simulink model "ThdRwLtStCshnFldIsPosChk1"  (R2024b)
settings: Solver=FixedStepDiscrete  StartTime=0.0  StopTime=10.0  FixedStep=0.01  RelTol=1e-3
undefined symbols (not defined in the file or in its folder): KeSMSuThrdRwCushFoldPosDelta_Val, KeSMSuThrdRwCushFoldPosTolr_Val
libraries: StIsPosChkLib x8, simulink x5
settings Model: Creator=sn2xws  LastModifiedBy=sn55gm
settings Model: ModifiedHistory=|
  | 2024.3.14
  | V2.3.0
  | Bug 813950 童锁Lock，Mode1_Easy Entry Mode 不应调用失败
  | 2024.6.25
  | V3.0.0 557模式流程V1.6
  | 2024.9.6 V3.0.1 新增Md56
  | 2024.10.14 V3.0.2 Md56使用的标定值修正
  | 2025.12.19 V3.8.0 Bug 991386 Md1 三排占座时未移动且报了成功
  | 2025.7.1 V3.13.0 新增MD61 MD62
settings SolverCC: AlgebraicLoopSolver=TrustRegion
settings DataIOCC: SaveFormat=StructureWithTime  ReturnWorkspaceOutputs=off
settings OptimizationCC: DefaultParameterBehavior=Inlined  EnhancedBackFolding=on  PassReuseOutputArgsAs=Individual arguments  ZeroExternalMemoryAtStartup=off  ZeroInternalMemoryAtStartup=off  OptimizeBlockOrder=speed  DifferentSizesBufferReuse=on  OptimizationCustomize=off  EfficientTunableParamExpr=on
settings DebuggingCC: ParameterTunabilityLossMsg=error  UnconnectedInputMsg=warning  UnconnectedOutputMsg=warning  UnconnectedLineMsg=warning  ArithmeticOperatorsInVariantConditions=warning
settings ModelReferenceCC: EnableRefExpFcnMdlSchedulingChecks=on  ModelReferenceNumInstancesAllowed=Single
settings SFSimCC: MATLABDynamicMemAlloc=off  CustomCodeUndefinedFunction=UseInterfaceOnly
settings RTWCC: Description=AUTOSAR  SystemTargetFile=autosar.tlc  GenCodeOnly=on  TemplateMakefile=ert_default_tmf  GenerateReport=on  IncludeHyperlinkInReport=on  LaunchReport=on  DataTypeReplacement=CDataTypesFixedWidth  GenerateTraceInfo=on  GenerateTraceReport=on  GenerateTraceReportSl=on  GenerateTraceReportSf=on  GenerateTraceReportEml=on  GPUComputeCapability=3.5
settings CodeAppCC: ForceParamTrailComments=on  IgnoreCustomStorageClasses=off  OperatorAnnotations=on  SimulinkDataObjDesc=on  SFDataObjDesc=on  InsertBlockDesc=on
settings STFCustomTargetCC: TargetLangStandard=C99 (ISO)  MultiwordLength=256  ParMdlRefBuildCompliant=on  CompOptLevelCompliant=on  IncludeMdlTerminateFcn=off  CombineOutputUpdateFcns=on  SuppressErrorStatus=on  ERTCustomFileBanners=on  SupportNonFinite=off  SupportComplex=off  SupportContinuousTime=off  SupportNonInlinedSFcns=off  RemoveResetFunc=on  MATLABClassNameForMDSCustomization=Simulink.SoftwareTarget.ERTCustomization  AutosarCompliant=on  UseToolchainInfoCompliant=on  LookupTableObjectStructAxisOrder=2,1,3,4,...  LUTObjectStructOrderEvenSpacing=Size,Table,Breakpoints  SystemTargetFile=autosar.tlc
settings ERTTargetCC: TargetLangStandard=C99 (ISO)  ConcurrentExecutionCompliant=off  IncludeMdlTerminateFcn=off  SuppressErrorStatus=on  SupportNonFinite=off  SupportComplex=off  ModelStepFunctionPrototypeControlCompliant=off  CPPClassGenCompliant=off  AutosarCompliant=on  LookupTableObjectStructAxisOrder=2,1,3,4,...  LUTObjectStructOrderEvenSpacing=Size,Table,Breakpoints  ERTCustomFileTemplate=example_file_process.tlc  ERTFilePackagingFormat=Compact  BooleanTrueId=TRUE  BooleanFalseId=FALSE  DynamicArrayContainerType=coder::array

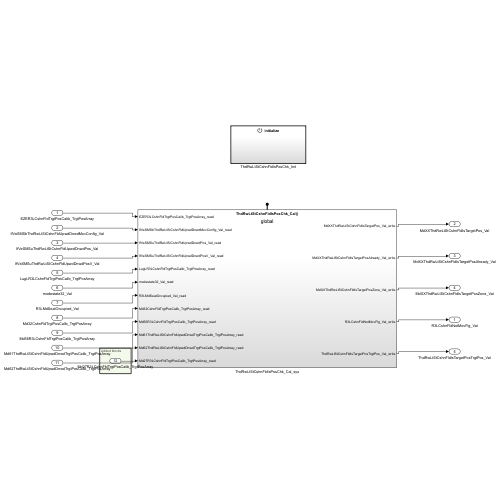
[thumbnail: Simulink's stored preview of the top-level diagram]
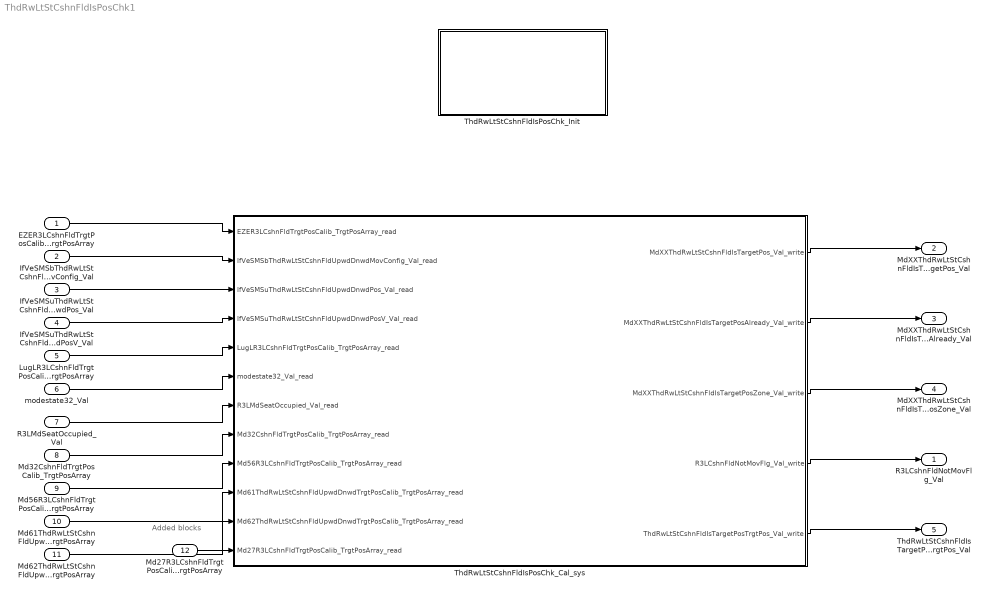
== system ThdRwLtStCshnFldIsPosChk1 ==
  note: Added blocks
  EZER3LCshnFldTrgtPosCalib_TrgtPosArray : Inport  Description=|  OutDataTypeStr=uint16  PortDimensions=3
      | 0:Pos
      | 1:Max
      | 2:Min
  IfVeSMSbThdRwLtStCshnFldUpwdDnwdMovConfig_Val : Inport  Port=2  OutDataTypeStr=boolean  PortDimensions=1
  IfVeSMSuThdRwLtStCshnFldUpwdDnwdPos_Val : Inport  Port=3  OutDataTypeStr=uint16  PortDimensions=1
  IfVeSMSuThdRwLtStCshnFldUpwdDnwdPosV_Val : Inport  Port=4  OutDataTypeStr=boolean  PortDimensions=1
  LugLR3LCshnFldTrgtPosCalib_TrgtPosArray : Inport  Description=|  Port=5  OutDataTypeStr=uint16  PortDimensions=3
      | 0:Pos
      | 1:Max
      | 2:Min
  modestate32_Val : Inport  Port=6  OutDataTypeStr=uint32  PortDimensions=1
  R3LMdSeatOccupied_Val : Inport  Port=7  OutDataTypeStr=boolean  PortDimensions=1
  Md32CshnFldTrgtPosCalib_TrgtPosArray : Inport  Description=|  Port=8  OutDataTypeStr=uint16  PortDimensions=3
      | 0:Pos
      | 1:Max
      | 2:Min
  Md56R3LCshnFldTrgtPosCalib_TrgtPosArray : Inport  Description=|  Port=9  OutDataTypeStr=uint16  PortDimensions=3
      | 0:Pos
      | 1:Max
      | 2:Min
  Md61ThdRwLtStCshnFldUpwdDnwdTrgtPosCalib_TrgtPosArray : Inport  Description=|  Port=10  OutDataTypeStr=uint16  PortDimensions=3
      | 0:Pos
      | 1:Max
      | 2:Min
  Md62ThdRwLtStCshnFldUpwdDnwdTrgtPosCalib_TrgtPosArray : Inport  Description=|  Port=11  OutDataTypeStr=uint16  PortDimensions=3
      | 0:Pos
      | 1:Max
      | 2:Min
  Md27R3LCshnFldTrgtPosCalib_TrgtPosArray : Inport  Description=|  Port=12  OutDataTypeStr=uint16  PortDimensions=3
      | 0:Pos
      | 1:Max
      | 2:Min
  ThdRwLtStCshnFldIsPosChk_Cal_sys : Subsystem
  ThdRwLtStCshnFldIsPosChk_Init : Subsystem
  R3LCshnFldNotMovFlg_Val : Outport  OutDataTypeStr=boolean  PortDimensions=1  VectorParamsAs1DForOutWhenUnconnected=off
  MdXXThdRwLtStCshnFldIsTargetPos_Val : Outport  Port=2  OutDataTypeStr=uint32  PortDimensions=1  VectorParamsAs1DForOutWhenUnconnected=off
  MdXXThdRwLtStCshnFldIsTargetPosAlready_Val : Outport  Port=3  OutDataTypeStr=uint32  PortDimensions=1  VectorParamsAs1DForOutWhenUnconnected=off
  MdXXThdRwLtStCshnFldIsTargetPosZone_Val : Outport  Port=4  OutDataTypeStr=uint32  PortDimensions=1  VectorParamsAs1DForOutWhenUnconnected=off
  ThdRwLtStCshnFldIsTargetPosTrgtPos_Val : Outport  Port=5  OutDataTypeStr=uint16  PortDimensions=1  VectorParamsAs1DForOutWhenUnconnected=off
  wires:
  EZER3LCshnFldTrgtPosCalib_TrgtPosArray/1 -> ThdRwLtStCshnFldIsPosChk_Cal_sys/1(EZER3LCshnFldTrgtPosCalib_TrgtPosArray_read)
  IfVeSMSbThdRwLtStCshnFldUpwdDnwdMovConfig_Val/1 -> ThdRwLtStCshnFldIsPosChk_Cal_sys/2(IfVeSMSbThdRwLtStCshnFldUpwdDnwdMovConfig_Val_read)
  IfVeSMSuThdRwLtStCshnFldUpwdDnwdPos_Val/1 -> ThdRwLtStCshnFldIsPosChk_Cal_sys/3(IfVeSMSuThdRwLtStCshnFldUpwdDnwdPos_Val_read)
  IfVeSMSuThdRwLtStCshnFldUpwdDnwdPosV_Val/1 -> ThdRwLtStCshnFldIsPosChk_Cal_sys/4(IfVeSMSuThdRwLtStCshnFldUpwdDnwdPosV_Val_read)
  LugLR3LCshnFldTrgtPosCalib_TrgtPosArray/1 -> ThdRwLtStCshnFldIsPosChk_Cal_sys/5(LugLR3LCshnFldTrgtPosCalib_TrgtPosArray_read)
  modestate32_Val/1 -> ThdRwLtStCshnFldIsPosChk_Cal_sys/6(modestate32_Val_read)
  ThdRwLtStCshnFldIsPosChk_Cal_sys/1(MdXXThdRwLtStCshnFldIsTargetPos_Val_write) -> MdXXThdRwLtStCshnFldIsTargetPos_Val/1
  ThdRwLtStCshnFldIsPosChk_Cal_sys/2(MdXXThdRwLtStCshnFldIsTargetPosAlready_Val_write) -> MdXXThdRwLtStCshnFldIsTargetPosAlready_Val/1
  ThdRwLtStCshnFldIsPosChk_Cal_sys/3(MdXXThdRwLtStCshnFldIsTargetPosZone_Val_write) -> MdXXThdRwLtStCshnFldIsTargetPosZone_Val/1
  ThdRwLtStCshnFldIsPosChk_Cal_sys/4(R3LCshnFldNotMovFlg_Val_write) -> R3LCshnFldNotMovFlg_Val/1
  ThdRwLtStCshnFldIsPosChk_Cal_sys/5(ThdRwLtStCshnFldIsTargetPosTrgtPos_Val_write) -> ThdRwLtStCshnFldIsTargetPosTrgtPos_Val/1
  R3LMdSeatOccupied_Val/1 -> ThdRwLtStCshnFldIsPosChk_Cal_sys/7(R3LMdSeatOccupied_Val_read)
  Md32CshnFldTrgtPosCalib_TrgtPosArray/1 -> ThdRwLtStCshnFldIsPosChk_Cal_sys/8(Md32CshnFldTrgtPosCalib_TrgtPosArray_read)
  Md56R3LCshnFldTrgtPosCalib_TrgtPosArray/1 -> ThdRwLtStCshnFldIsPosChk_Cal_sys/9(Md56R3LCshnFldTrgtPosCalib_TrgtPosArray_read)
  Md61ThdRwLtStCshnFldUpwdDnwdTrgtPosCalib_TrgtPosArray/1 -> ThdRwLtStCshnFldIsPosChk_Cal_sys/10(Md61ThdRwLtStCshnFldUpwdDnwdTrgtPosCalib_TrgtPosArray_read)
  Md62ThdRwLtStCshnFldUpwdDnwdTrgtPosCalib_TrgtPosArray/1 -> ThdRwLtStCshnFldIsPosChk_Cal_sys/11(Md62ThdRwLtStCshnFldUpwdDnwdTrgtPosCalib_TrgtPosArray_read)
  Md27R3LCshnFldTrgtPosCalib_TrgtPosArray/1 -> ThdRwLtStCshnFldIsPosChk_Cal_sys/12(Md27R3LCshnFldTrgtPosCalib_TrgtPosArray_read)

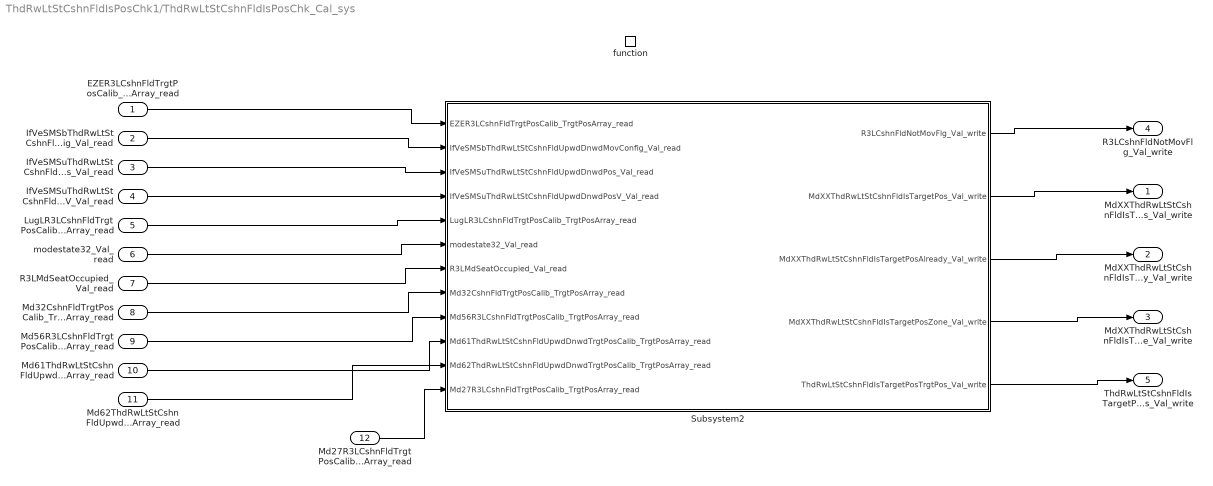
== system ThdRwLtStCshnFldIsPosChk1/ThdRwLtStCshnFldIsPosChk_Cal_sys ==
  EZER3LCshnFldTrgtPosCalib_TrgtPosArray_read : Inport
  IfVeSMSbThdRwLtStCshnFldUpwdDnwdMovConfig_Val_read : Inport  Port=2
  IfVeSMSuThdRwLtStCshnFldUpwdDnwdPos_Val_read : Inport  Port=3
  IfVeSMSuThdRwLtStCshnFldUpwdDnwdPosV_Val_read : Inport  Port=4
  LugLR3LCshnFldTrgtPosCalib_TrgtPosArray_read : Inport  Port=5
  modestate32_Val_read : Inport  Port=6
  R3LMdSeatOccupied_Val_read : Inport  Port=7
  Md32CshnFldTrgtPosCalib_TrgtPosArray_read : Inport  Port=8
  Md56R3LCshnFldTrgtPosCalib_TrgtPosArray_read : Inport  Port=9
  Md61ThdRwLtStCshnFldUpwdDnwdTrgtPosCalib_TrgtPosArray_read : Inport  Port=10
  Md62ThdRwLtStCshnFldUpwdDnwdTrgtPosCalib_TrgtPosArray_read : Inport  Port=11
  Md27R3LCshnFldTrgtPosCalib_TrgtPosArray_read : Inport  Port=12
  function : TriggerPort  TriggerType=function-call  IsSimulinkFunction=on  FunctionName=ThdRwLtStCshnFldIsPosChk_Cal  VariantControl=(inherit)
  Subsystem2 : Subsystem
  MdXXThdRwLtStCshnFldIsTargetPos_Val_write : Outport  VectorParamsAs1DForOutWhenUnconnected=off
      settings: EnsureOutportIsVirtual=on
  MdXXThdRwLtStCshnFldIsTargetPosAlready_Val_write : Outport  Port=2  VectorParamsAs1DForOutWhenUnconnected=off
      settings: EnsureOutportIsVirtual=on
  MdXXThdRwLtStCshnFldIsTargetPosZone_Val_write : Outport  Port=3  VectorParamsAs1DForOutWhenUnconnected=off
      settings: EnsureOutportIsVirtual=on
  R3LCshnFldNotMovFlg_Val_write : Outport  Port=4  VectorParamsAs1DForOutWhenUnconnected=off
      settings: EnsureOutportIsVirtual=on
  ThdRwLtStCshnFldIsTargetPosTrgtPos_Val_write : Outport  Port=5  VectorParamsAs1DForOutWhenUnconnected=off
      settings: EnsureOutportIsVirtual=on
  wires:
  Subsystem2/1(R3LCshnFldNotMovFlg_Val_write) -> R3LCshnFldNotMovFlg_Val_write/1
  Subsystem2/2(MdXXThdRwLtStCshnFldIsTargetPos_Val_write) -> MdXXThdRwLtStCshnFldIsTargetPos_Val_write/1
  Subsystem2/3(MdXXThdRwLtStCshnFldIsTargetPosAlready_Val_write) -> MdXXThdRwLtStCshnFldIsTargetPosAlready_Val_write/1
  Subsystem2/4(MdXXThdRwLtStCshnFldIsTargetPosZone_Val_write) -> MdXXThdRwLtStCshnFldIsTargetPosZone_Val_write/1
  Subsystem2/5(ThdRwLtStCshnFldIsTargetPosTrgtPos_Val_write) -> ThdRwLtStCshnFldIsTargetPosTrgtPos_Val_write/1
  EZER3LCshnFldTrgtPosCalib_TrgtPosArray_read/1 -> Subsystem2/1(EZER3LCshnFldTrgtPosCalib_TrgtPosArray_read)
  IfVeSMSbThdRwLtStCshnFldUpwdDnwdMovConfig_Val_read/1 -> Subsystem2/2(IfVeSMSbThdRwLtStCshnFldUpwdDnwdMovConfig_Val_read)
  IfVeSMSuThdRwLtStCshnFldUpwdDnwdPos_Val_read/1 -> Subsystem2/3(IfVeSMSuThdRwLtStCshnFldUpwdDnwdPos_Val_read)
  IfVeSMSuThdRwLtStCshnFldUpwdDnwdPosV_Val_read/1 -> Subsystem2/4(IfVeSMSuThdRwLtStCshnFldUpwdDnwdPosV_Val_read)
  LugLR3LCshnFldTrgtPosCalib_TrgtPosArray_read/1 -> Subsystem2/5(LugLR3LCshnFldTrgtPosCalib_TrgtPosArray_read)
  modestate32_Val_read/1 -> Subsystem2/6(modestate32_Val_read)
  R3LMdSeatOccupied_Val_read/1 -> Subsystem2/7(R3LMdSeatOccupied_Val_read)
  Md32CshnFldTrgtPosCalib_TrgtPosArray_read/1 -> Subsystem2/8(Md32CshnFldTrgtPosCalib_TrgtPosArray_read)
  Md56R3LCshnFldTrgtPosCalib_TrgtPosArray_read/1 -> Subsystem2/9(Md56R3LCshnFldTrgtPosCalib_TrgtPosArray_read)
  Md61ThdRwLtStCshnFldUpwdDnwdTrgtPosCalib_TrgtPosArray_read/1 -> Subsystem2/10(Md61ThdRwLtStCshnFldUpwdDnwdTrgtPosCalib_TrgtPosArray_read)
  Md62ThdRwLtStCshnFldUpwdDnwdTrgtPosCalib_TrgtPosArray_read/1 -> Subsystem2/11(Md62ThdRwLtStCshnFldUpwdDnwdTrgtPosCalib_TrgtPosArray_read)
  Md27R3LCshnFldTrgtPosCalib_TrgtPosArray_read/1 -> Subsystem2/12(Md27R3LCshnFldTrgtPosCalib_TrgtPosArray_read)

== system ThdRwLtStCshnFldIsPosChk1/ThdRwLtStCshnFldIsPosChk_Init ==
  Event Listener : EventListener  EventName=reset
  PA_KeSMSuThrdRwCushFoldPosDelta_Val : Constant  Value=KeSMSuThrdRwCushFoldPosDelta_Val
  PA_KeSMSuThrdRwCushFoldPosTolr_Val : Constant  Value=KeSMSuThrdRwCushFoldPosTolr_Val
  Terminator_1 : Terminator
  Terminator_2 : Terminator
  wires:
  PA_KeSMSuThrdRwCushFoldPosDelta_Val/1 -> Terminator_1/1
  PA_KeSMSuThrdRwCushFoldPosTolr_Val/1 -> Terminator_2/1

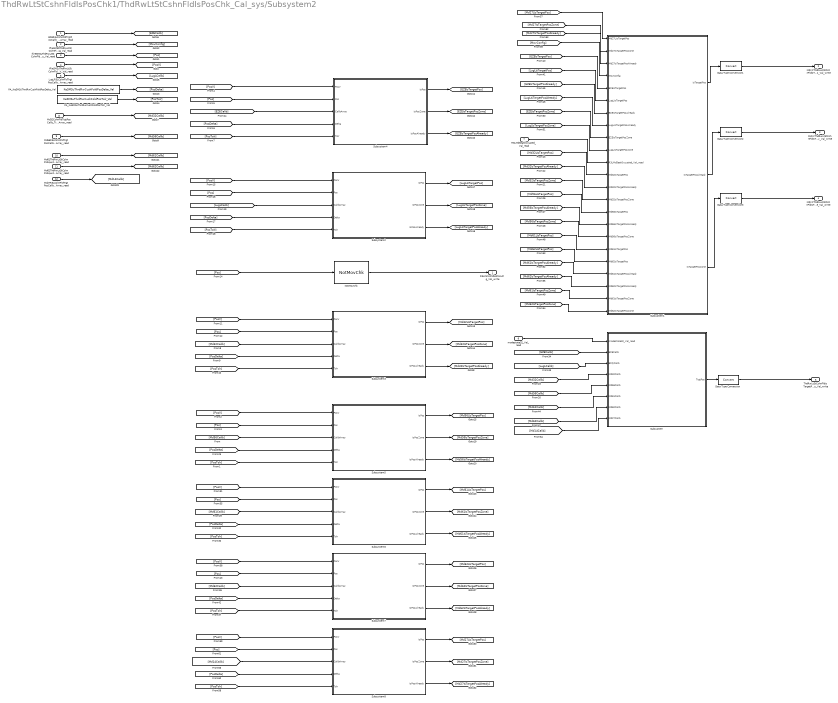
== system ThdRwLtStCshnFldIsPosChk1/ThdRwLtStCshnFldIsPosChk_Cal_sys/Subsystem2 ==
  EZER3LCshnFldTrgtPosCalib_TrgtPosArray_read : Inport
  IfVeSMSbThdRwLtStCshnFldUpwdDnwdMovConfig_Val_read : Inport  Port=2
  IfVeSMSuThdRwLtStCshnFldUpwdDnwdPos_Val_read : Inport  Port=3
  IfVeSMSuThdRwLtStCshnFldUpwdDnwdPosV_Val_read : Inport  Port=4
  LugLR3LCshnFldTrgtPosCalib_TrgtPosArray_read : Inport  Port=5
  modestate32_Val_read : Inport  Port=6
  R3LMdSeatOccupied_Val_read : Inport  Port=7
  Md32CshnFldTrgtPosCalib_TrgtPosArray_read : Inport  Port=8
  Md56R3LCshnFldTrgtPosCalib_TrgtPosArray_read : Inport  Port=9
  Md61ThdRwLtStCshnFldUpwdDnwdTrgtPosCalib_TrgtPosArray_read : Inport  Port=10
  Md62ThdRwLtStCshnFldUpwdDnwdTrgtPosCalib_TrgtPosArray_read : Inport  Port=11
  Md27R3LCshnFldTrgtPosCalib_TrgtPosArray_read : Inport  Port=12
  Data Type Conversion{,1..3} (4 alike) : DataTypeConversion  SaturateOnIntegerOverflow=off  RndMeth=Floor
  NotMovChk : StIsPosChkLib/NotMovChk  SystemSampleTime=-1  VariantActivationTime=update diagram  AllowFlexibleInterface=on  Latency=0  AutoFrameSizeCalculation=off
  PA_KeSMSuThrdRwCushFoldPosDelta_Val : Constant  Value=KeSMSuThrdRwCushFoldPosDelta_Val
  PA_KeSMSuThrdRwCushFoldPosTolr_Val : Constant  Value=KeSMSuThrdRwCushFoldPosTolr_Val
  Subsystem : Subsystem
  Subsystem1 : Subsystem
  Subsystem2 : Subsystem
  Subsystem3 : Subsystem
  Subsystem4 : Subsystem
  Subsystem5 : Subsystem
  Subsystem6 : Subsystem
  Subsystem7 : Subsystem
  Subsystem8 : Subsystem
  R3LCshnFldNotMovFlg_Val_write : Outport  VectorParamsAs1DForOutWhenUnconnected=off
      settings: EnsureOutportIsVirtual=on
  MdXXThdRwLtStCshnFldIsTargetPos_Val_write : Outport  Port=2  VectorParamsAs1DForOutWhenUnconnected=off
      settings: EnsureOutportIsVirtual=on
  MdXXThdRwLtStCshnFldIsTargetPosAlready_Val_write : Outport  Port=3  VectorParamsAs1DForOutWhenUnconnected=off
      settings: EnsureOutportIsVirtual=on
  MdXXThdRwLtStCshnFldIsTargetPosZone_Val_write : Outport  Port=4  VectorParamsAs1DForOutWhenUnconnected=off
      settings: EnsureOutportIsVirtual=on
  ThdRwLtStCshnFldIsTargetPosTrgtPos_Val_write : Outport  Port=5  VectorParamsAs1DForOutWhenUnconnected=off
      settings: EnsureOutportIsVirtual=on
  wires:
  [LugLCalib] -> Subsystem2/3(CalibArray)
  [Pos] -> Subsystem4/2(Pos)
  [PosTolr] -> Subsystem2/5(Tolr)
  modestate32_Val_read/1 -> Subsystem/1(modestate32_Val_read)
  Subsystem/1(TrgtPos) -> Data Type Conversion/1
  Subsystem4/2(IsPosZone) -> [EZEIsTargetPosZone]
  [PosDelta] -> Subsystem2/4(Delta)
  Data Type Conversion/1 -> ThdRwLtStCshnFldIsTargetPosTrgtPos_Val_write/1
  NotMovChk/1 -> R3LCshnFldNotMovFlg_Val_write/1
  Subsystem4/3(IsPosAlready) -> [EZEIsTargetPosAlready]
  [LugLIsTargetPos] -> Subsystem1/6(LugLIsTargetPos)
  Subsystem1/3(IsTargetPosZone) -> Data Type Conversion3/1
  [LugLIsTargetPosZone] -> Subsystem1/10(LugLIsTargetPosZone)
  [PosDelta] -> Subsystem4/4(Delta)
  [MovConfig] -> Subsystem1/4(MovConfig)
  Subsystem4/1(IsPos) -> [EZEIsTargetPos]
  Subsystem1/2(IsTargetPosAlready) -> Data Type Conversion2/1
  PA_KeSMSuThrdRwCushFoldPosDelta_Val/1 -> [PosDelta]
  Data Type Conversion2/1 -> MdXXThdRwLtStCshnFldIsTargetPosAlready_Val_write/1
  PA_KeSMSuThrdRwCushFoldPosTolr_Val/1 -> [PosTolr]
  IfVeSMSuThdRwLtStCshnFldUpwdDnwdPos_Val_read/1 -> [Pos]
  Subsystem2/1(IsPos) -> [LugLIsTargetPos]
  IfVeSMSuThdRwLtStCshnFldUpwdDnwdPosV_Val_read/1 -> [PosV]
  [PosV] -> Subsystem4/1(PosV)
  [PosV] -> Subsystem2/1(PosV)
  [Pos] -> Subsystem2/2(Pos)
  [PosTolr] -> Subsystem4/5(Tolr)
  Subsystem2/2(IsPosZone) -> [LugLIsTargetPosZone]
  Subsystem1/1(IsTargetPos) -> Data Type Conversion1/1
  LugLR3LCshnFldTrgtPosCalib_TrgtPosArray_read/1 -> [LugLCalib]
  Subsystem2/3(IsPosAlready) -> [LugLIsTargetPosAlready]
  Data Type Conversion3/1 -> MdXXThdRwLtStCshnFldIsTargetPosZone_Val_write/1
  [LugLCalib] -> Subsystem/3(EZQCalib)
  [LugLIsTargetPosAlready] -> Subsystem1/8(LugLIsTargetPosAlready)
  [EZEIsTargetPosZone] -> Subsystem1/9(EZEIsTargetPosZone)
  IfVeSMSbThdRwLtStCshnFldUpwdDnwdMovConfig_Val_read/1 -> [MovConfig]
  [EZECalib] -> Subsystem4/3(CalibArray)
  [EZECalib] -> Subsystem/2(EZECalib)
  EZER3LCshnFldTrgtPosCalib_TrgtPosArray_read/1 -> [EZECalib]
  Data Type Conversion1/1 -> MdXXThdRwLtStCshnFldIsTargetPos_Val_write/1
  [Pos] -> NotMovChk/1
  [EZEIsTargetPosAlready] -> Subsystem1/7(EZEIsTargetPosAlready)
  [EZEIsTargetPos] -> Subsystem1/5(EZEIsTargetPos)
  R3LMdSeatOccupied_Val_read/1 -> Subsystem1/11(R3LMdSeatOccupied_Val_read)
  Md32CshnFldTrgtPosCalib_TrgtPosArray_read/1 -> [Md32Calib]
  [Md32Calib] -> Subsystem3/3(CalibArray)
  [PosDelta] -> Subsystem3/4(Delta)
  [PosTolr] -> Subsystem3/5(Tolr)
  [Pos] -> Subsystem3/2(Pos)
  [PosV] -> Subsystem3/1(PosV)
  Subsystem3/3(IsPosAlready) -> [Md32IsTargetPosAlready]
  Subsystem3/2(IsPosZone) -> [Md32IsTargetPosZone]
  Subsystem3/1(IsPos) -> [Md32LIsTargetPos]
  [Md32Calib] -> Subsystem/4(Md32Calib)
  [Md32LIsTargetPos] -> Subsystem1/12(Md32IsTargetPos)
  [Md32IsTargetPosZone] -> Subsystem1/14(Md32IsTargetPosZone)
  [Md32IsTargetPosAlready] -> Subsystem1/13(Md32IsTargetPosAlready)
  Md56R3LCshnFldTrgtPosCalib_TrgtPosArray_read/1 -> [Md56Calib]
  [PosV] -> Subsystem5/1(PosV)
  [Pos] -> Subsystem5/2(Pos)
  [PosTolr] -> Subsystem5/5(Tolr)
  [PosDelta] -> Subsystem5/4(Delta)
  [Md56Calib] -> Subsystem5/3(CalibArray)
  Subsystem5/1(IsPos) -> [Md56LIsTargetPos]
  Subsystem5/2(IsPosZone) -> [Md56IsTargetPosZone]
  Subsystem5/3(IsPosAlready) -> [Md56IsTargetPosAlready]
  [Md56Calib] -> Subsystem/5(Md56Calib)
  [Md56IsTargetPosZone] -> Subsystem1/17(Md56IsTargetPosZone)
  [Md56IsTargetPosAlready] -> Subsystem1/16(Md56IsTargetPosAlready)
  [Md56LIsTargetPos] -> Subsystem1/15(Md56IsTargetPos)
  Md61ThdRwLtStCshnFldUpwdDnwdTrgtPosCalib_TrgtPosArray_read/1 -> [Md61Calib]
  Md62ThdRwLtStCshnFldUpwdDnwdTrgtPosCalib_TrgtPosArray_read/1 -> [Md62Calib]
  Subsystem6/3(IsPosAlready) -> [Md61IsTargetPosAlready]
  Subsystem6/2(IsPosZone) -> [Md61IsTargetPosZone]
  Subsystem6/1(IsPos) -> [Md61LIsTargetPos]
  [Md61Calib] -> Subsystem6/3(CalibArray)
  [PosDelta] -> Subsystem6/4(Delta)
  [PosTolr] -> Subsystem6/5(Tolr)
  [Pos] -> Subsystem6/2(Pos)
  [PosV] -> Subsystem6/1(PosV)
  [PosV] -> Subsystem7/1(PosV)
  [Pos] -> Subsystem7/2(Pos)
  [PosTolr] -> Subsystem7/5(Tolr)
  [PosDelta] -> Subsystem7/4(Delta)
  [Md62Calib] -> Subsystem7/3(CalibArray)
  Subsystem7/1(IsPos) -> [Md62LIsTargetPos]
  Subsystem7/2(IsPosZone) -> [Md62IsTargetPosZone]
  Subsystem7/3(IsPosAlready) -> [Md62IsTargetPosAlready]
  [Md61Calib] -> Subsystem/6(Md61Calib)
  [Md62Calib] -> Subsystem/7(Md62Calib)
  [Md61LIsTargetPos] -> Subsystem1/18(Md61IsTargetPos)
  [Md62LIsTargetPos] -> Subsystem1/19(Md62IsTargetPos)
  [Md61IsTargetPosAlready] -> Subsystem1/20(Md61IsTargetPosAlready)
  [Md62IsTargetPosAlready] -> Subsystem1/21(Md62IsTargetPosAlready)
  [Md62IsTargetPosZone] -> Subsystem1/23(Md62IsTargetPosZone)
  [Md61IsTargetPosZone] -> Subsystem1/22(Md61IsTargetPosZone)
  Md27R3LCshnFldTrgtPosCalib_TrgtPosArray_read/1 -> [Md14Calib]
  Subsystem8/3(IsPosAlready) -> [Md27IsTargetPosAlready]
  [Md14Calib] -> Subsystem8/3(CalibArray)
  Subsystem8/1(IsPos) -> [Md27LIsTargetPos]
  [Pos] -> Subsystem8/2(Pos)
  [PosDelta] -> Subsystem8/4(Delta)
  [PosV] -> Subsystem8/1(PosV)
  Subsystem8/2(IsPosZone) -> [Md27IsTargetPosZone]
  [PosTolr] -> Subsystem8/5(Tolr)
  [Md27LIsTargetPos] -> Subsystem1/1(Md27LIsTargetPos)
  [Md27IsTargetPosZone] -> Subsystem1/2(Md27IsTargetPosZone)
  [Md27IsTargetPosAlready] -> Subsystem1/3(Md27IsTargetPosAlready)
  [Md14Calib] -> Subsystem/8(Md27Calib)

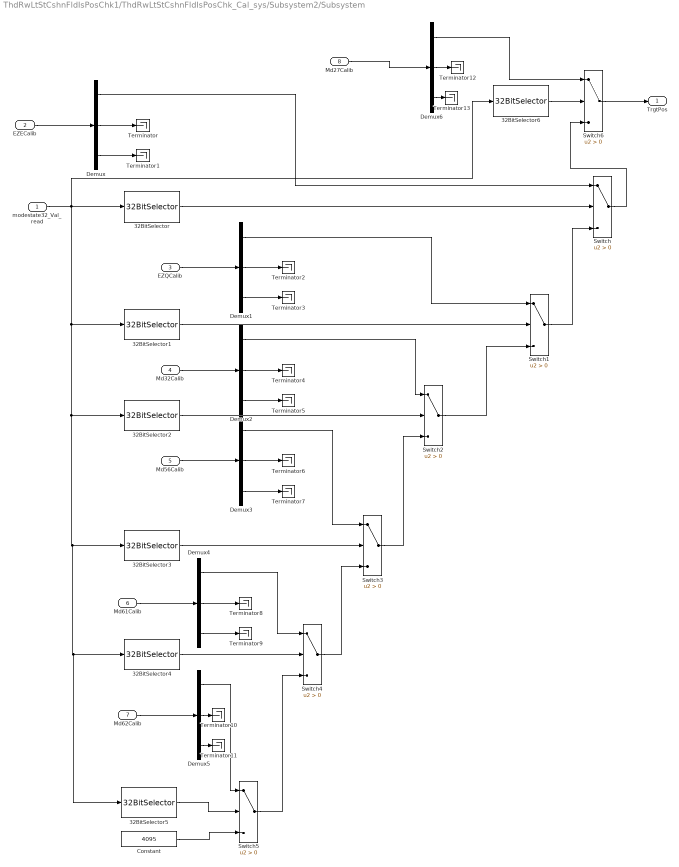
== system ThdRwLtStCshnFldIsPosChk1/ThdRwLtStCshnFldIsPosChk_Cal_sys/Subsystem2/Subsystem ==
  modestate32_Val_read : Inport
  EZECalib : Inport  Port=2
  EZQCalib : Inport  Port=3
  Md32Calib : Inport  Port=4
  Md56Calib : Inport  Port=5
  Md61Calib : Inport  Port=6
  Md62Calib : Inport  Port=7
  Md27Calib : Inport  Port=8
  32BitSelector : StIsPosChkLib/32BitSelector  BitNum=0
  32BitSelector1 : StIsPosChkLib/32BitSelector  BitNum=7
  32BitSelector2 : StIsPosChkLib/32BitSelector  BitNum=31
  32BitSelector3 : StIsPosChkLib/32BitSelector  BitNum=24
  32BitSelector4 : StIsPosChkLib/32BitSelector  BitNum=5
  32BitSelector5 : StIsPosChkLib/32BitSelector  BitNum=6
  32BitSelector6 : StIsPosChkLib/32BitSelector  BitNum=13
  Constant : Constant  Value=4095  OutDataTypeStr=uint16
  Demux{,1..6} (7 alike) : Demux  Outputs=3
  Switch{,1..6} (7 alike) : Switch  Criteria=u2 > Threshold  SaturateOnIntegerOverflow=off  InputSameDT=off
  Terminator{,1..13} (14 alike) : Terminator
  TrgtPos : Outport  VectorParamsAs1DForOutWhenUnconnected=off
      settings: EnsureOutportIsVirtual=on
  wires:
  32BitSelector/1 -> Switch/2
  modestate32_Val_read/1 -> 32BitSelector6/1, 32BitSelector5/1, 32BitSelector4/1, 32BitSelector3/1, 32BitSelector2/1, 32BitSelector1/1, 32BitSelector/1
  Demux/1 -> Switch/1
  Demux/3 -> Terminator1/1
  Demux/2 -> Terminator/1
  EZECalib/1 -> Demux/1
  EZQCalib/1 -> Demux1/1
  Demux1/2 -> Terminator2/1
  Demux1/3 -> Terminator3/1
  Demux1/1 -> Switch1/1
  Switch1/1 -> Switch/3
  32BitSelector1/1 -> Switch1/2
  Switch2/1 -> Switch1/3
  32BitSelector2/1 -> Switch2/2
  Demux2/1 -> Switch2/1
  Demux2/3 -> Terminator5/1
  Demux2/2 -> Terminator4/1
  Md32Calib/1 -> Demux2/1
  Md56Calib/1 -> Demux3/1
  Demux3/2 -> Terminator6/1
  Demux3/1 -> Switch3/1
  Switch3/1 -> Switch2/3
  32BitSelector3/1 -> Switch3/2
  Demux3/3 -> Terminator7/1
  Switch4/1 -> Switch3/3
  32BitSelector4/1 -> Switch4/2
  Switch5/1 -> Switch4/3
  32BitSelector5/1 -> Switch5/2
  Demux4/3 -> Terminator9/1
  Demux4/2 -> Terminator8/1
  Md61Calib/1 -> Demux4/1
  Demux4/1 -> Switch4/1
  Md62Calib/1 -> Demux5/1
  Demux5/3 -> Terminator11/1
  Demux5/2 -> Terminator10/1
  Demux5/1 -> Switch5/1
  32BitSelector6/1 -> Switch6/2
  Demux6/1 -> Switch6/1
  Demux6/3 -> Terminator13/1
  Demux6/2 -> Terminator12/1
  Md27Calib/1 -> Demux6/1
  Constant/1 -> Switch5/3
  Switch/1 -> Switch6/3
  Switch6/1 -> TrgtPos/1

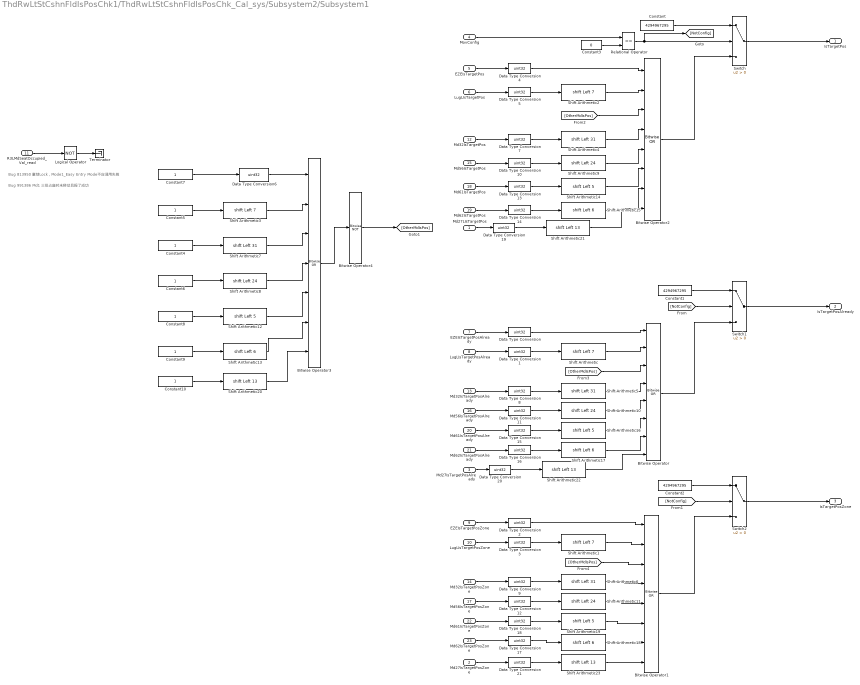
== system ThdRwLtStCshnFldIsPosChk1/ThdRwLtStCshnFldIsPosChk_Cal_sys/Subsystem2/Subsystem1 ==
  note: Bug 991386 Md1 三排占座时未移动且报了成功
  note: Bug 813950 童锁Lock，Mode1_Easy Entry Mode 不应调用失败
  Md27LIsTargetPos : Inport
  Md27IsTargetPosZone : Inport  Port=2
  Md27IsTargetPosAlready : Inport  Port=3
  MovConfig : Inport  Port=4
  EZEIsTargetPos : Inport  Port=5
  LugLIsTargetPos : Inport  Port=6
  EZEIsTargetPosAlready : Inport  Port=7
  LugLIsTargetPosAlready : Inport  Port=8
  EZEIsTargetPosZone : Inport  Port=9
  LugLIsTargetPosZone : Inport  Port=10
  R3LMdSeatOccupied_Val_read : Inport  Port=11
  Md32IsTargetPos : Inport  Port=12
  Md32IsTargetPosAlready : Inport  Port=13
  Md32IsTargetPosZone : Inport  Port=14
  Md56IsTargetPos : Inport  Port=15
  Md56IsTargetPosAlready : Inport  Port=16
  Md56IsTargetPosZone : Inport  Port=17
  Md61IsTargetPos : Inport  Port=18
  Md62IsTargetPos : Inport  Port=19
  Md61IsTargetPosAlready : Inport  Port=20
  Md62IsTargetPosAlready : Inport  Port=21
  Md61IsTargetPosZone : Inport  Port=22
  Md62IsTargetPosZone : Inport  Port=23
  Bitwise Operator : simulink/Logic and Bit Operations/Bitwise Operator  logicop=OR  UseBitMask=off  NumInputPorts=8  BitMask=bin2dec('11011001')  BitMaskRealWorld=Stored Integer
  Bitwise Operator1 : simulink/Logic and Bit Operations/Bitwise Operator  logicop=OR  UseBitMask=off  NumInputPorts=8  BitMask=bin2dec('11011001')  BitMaskRealWorld=Stored Integer
  Bitwise Operator2 : simulink/Logic and Bit Operations/Bitwise Operator  logicop=OR  UseBitMask=off  NumInputPorts=8  BitMask=bin2dec('11011001')  BitMaskRealWorld=Stored Integer
  Bitwise Operator3 : simulink/Logic and Bit Operations/Bitwise Operator  logicop=OR  UseBitMask=off  NumInputPorts=7  BitMask=bin2dec('11011001')  BitMaskRealWorld=Stored Integer
  Bitwise Operator4 : simulink/Logic and Bit Operations/Bitwise Operator  logicop=NOT  UseBitMask=off  BitMask=bin2dec('11011001')  BitMaskRealWorld=Stored Integer
  Constant : Constant  Value=4294967295  OutDataTypeStr=uint32
  Constant1 : Constant  Value=4294967295  OutDataTypeStr=uint32
  Constant{4..10} (7 alike) : Constant  OutDataTypeStr=uint32
  Constant2 : Constant  Value=4294967295  OutDataTypeStr=uint32
  Constant3 : Constant  Value=0  OutDataTypeStr=uint8
  Data Type Conversion{,1..21} (22 alike) : DataTypeConversion  OutDataTypeStr=uint32  SaturateOnIntegerOverflow=off  RndMeth=Floor
  Logical Operator : Logic  Operator=NOT  AllPortsSameDT=off  OutDataTypeStr=boolean
  Relational Operator : RelationalOperator  Operator===  OutDataTypeStr=boolean  RndMeth=Simplest  InputSameDT=off
  Shift Arithmetic{,1..3} (4 alike) : ArithShift  BitShiftNumber=7  BitShiftDirection=Left
  Shift Arithmetic{8..11} (4 alike) : ArithShift  BitShiftNumber=24  BitShiftDirection=Left
  Shift Arithmetic{12,14,16,19} (4 alike) : ArithShift  BitShiftNumber=5  BitShiftDirection=Left
  Shift Arithmetic{13,15,17..18} (4 alike) : ArithShift  BitShiftNumber=6  BitShiftDirection=Left
  Shift Arithmetic{20..23} (4 alike) : ArithShift  BitShiftNumber=13  BitShiftDirection=Left
  Shift Arithmetic{4..7} (4 alike) : ArithShift  BitShiftNumber=31  BitShiftDirection=Left
  Switch : Switch  Criteria=u2 > Threshold  SaturateOnIntegerOverflow=off  InputSameDT=off
  Switch1 : Switch  Criteria=u2 > Threshold  SaturateOnIntegerOverflow=off  InputSameDT=off
  Switch2 : Switch  Criteria=u2 > Threshold  SaturateOnIntegerOverflow=off  InputSameDT=off
  Terminator : Terminator
  IsTargetPos : Outport  VectorParamsAs1DForOutWhenUnconnected=off
      settings: EnsureOutportIsVirtual=on
  IsTargetPosAlready : Outport  Port=2  VectorParamsAs1DForOutWhenUnconnected=off
      settings: EnsureOutportIsVirtual=on
  IsTargetPosZone : Outport  Port=3  VectorParamsAs1DForOutWhenUnconnected=off
      settings: EnsureOutportIsVirtual=on
  wires:
  Constant3/1 -> Relational Operator/2
  Constant/1 -> Switch/1
  Relational Operator/1 -> [NotConfig], Switch/2
  MovConfig/1 -> Relational Operator/1
  Switch/1 -> IsTargetPos/1
  [NotConfig] -> Switch1/2
  Constant1/1 -> Switch1/1
  Switch1/1 -> IsTargetPosAlready/1
  Switch2/1 -> IsTargetPosZone/1
  Constant2/1 -> Switch2/1
  [NotConfig] -> Switch2/2
  Data Type Conversion1/1 -> Shift Arithmetic/1
  Data Type Conversion/1 -> Bitwise Operator/1
  Shift Arithmetic/1 -> Bitwise Operator/2
  Shift Arithmetic1/1 -> Bitwise Operator1/2
  Data Type Conversion2/1 -> Bitwise Operator1/1
  Data Type Conversion3/1 -> Shift Arithmetic1/1
  Bitwise Operator1/1 -> Switch2/3
  Bitwise Operator/1 -> Switch1/3
  Shift Arithmetic2/1 -> Bitwise Operator2/2
  Data Type Conversion4/1 -> Bitwise Operator2/1
  Data Type Conversion5/1 -> Shift Arithmetic2/1
  Bitwise Operator2/1 -> Switch/3
  EZEIsTargetPos/1 -> Data Type Conversion4/1
  LugLIsTargetPos/1 -> Data Type Conversion5/1
  LugLIsTargetPosZone/1 -> Data Type Conversion3/1
  EZEIsTargetPosZone/1 -> Data Type Conversion2/1
  LugLIsTargetPosAlready/1 -> Data Type Conversion1/1
  EZEIsTargetPosAlready/1 -> Data Type Conversion/1
  Shift Arithmetic3/1 -> Bitwise Operator3/2
  Constant5/1 -> Shift Arithmetic3/1
  Bitwise Operator3/1 -> Bitwise Operator4/1
  Bitwise Operator4/1 -> [OtherMdIsPos]
  [OtherMdIsPos] -> Bitwise Operator2/3
  [OtherMdIsPos] -> Bitwise Operator/3
  [OtherMdIsPos] -> Bitwise Operator1/3
  Data Type Conversion6/1 -> Bitwise Operator3/1
  R3LMdSeatOccupied_Val_read/1 -> Logical Operator/1
  Md32IsTargetPos/1 -> Data Type Conversion7/1
  Data Type Conversion7/1 -> Shift Arithmetic4/1
  Shift Arithmetic4/1 -> Bitwise Operator2/4
  Md32IsTargetPosAlready/1 -> Data Type Conversion8/1
  Data Type Conversion8/1 -> Shift Arithmetic5/1
  Shift Arithmetic5/1 -> Bitwise Operator/4
  Md32IsTargetPosZone/1 -> Data Type Conversion9/1
  Data Type Conversion9/1 -> Shift Arithmetic6/1
  Shift Arithmetic6/1 -> Bitwise Operator1/4
  Constant4/1 -> Shift Arithmetic7/1
  Shift Arithmetic7/1 -> Bitwise Operator3/3
  Constant6/1 -> Shift Arithmetic8/1
  Shift Arithmetic8/1 -> Bitwise Operator3/4
  Shift Arithmetic9/1 -> Bitwise Operator2/5
  Data Type Conversion10/1 -> Shift Arithmetic9/1
  Md56IsTargetPos/1 -> Data Type Conversion10/1
  Shift Arithmetic10/1 -> Bitwise Operator/5
  Data Type Conversion11/1 -> Shift Arithmetic10/1
  Md56IsTargetPosAlready/1 -> Data Type Conversion11/1
  Shift Arithmetic11/1 -> Bitwise Operator1/5
  Data Type Conversion12/1 -> Shift Arithmetic11/1
  Md56IsTargetPosZone/1 -> Data Type Conversion12/1
  Constant7/1 -> Data Type Conversion6/1
  Logical Operator/1 -> Terminator/1
  Constant8/1 -> Shift Arithmetic12/1
  Constant9/1 -> Shift Arithmetic13/1
  Shift Arithmetic12/1 -> Bitwise Operator3/5
  Shift Arithmetic13/1 -> Bitwise Operator3/6
  Md61IsTargetPos/1 -> Data Type Conversion13/1
  Data Type Conversion13/1 -> Shift Arithmetic14/1
  Shift Arithmetic14/1 -> Bitwise Operator2/6
  Shift Arithmetic15/1 -> Bitwise Operator2/7
  Data Type Conversion14/1 -> Shift Arithmetic15/1
  Md62IsTargetPos/1 -> Data Type Conversion14/1
  Md61IsTargetPosAlready/1 -> Data Type Conversion15/1
  Data Type Conversion15/1 -> Shift Arithmetic16/1
  Shift Arithmetic16/1 -> Bitwise Operator/6
  Shift Arithmetic17/1 -> Bitwise Operator/7
  Data Type Conversion16/1 -> Shift Arithmetic17/1
  Md62IsTargetPosAlready/1 -> Data Type Conversion16/1
  Md62IsTargetPosZone/1 -> Data Type Conversion17/1
  Data Type Conversion17/1 -> Shift Arithmetic18/1
  Shift Arithmetic18/1 -> Bitwise Operator1/7
  Shift Arithmetic19/1 -> Bitwise Operator1/6
  Data Type Conversion18/1 -> Shift Arithmetic19/1
  Md61IsTargetPosZone/1 -> Data Type Conversion18/1
  Constant10/1 -> Shift Arithmetic20/1
  Shift Arithmetic20/1 -> Bitwise Operator3/7
  Shift Arithmetic21/1 -> Bitwise Operator2/8
  Data Type Conversion19/1 -> Shift Arithmetic21/1
  Md27LIsTargetPos/1 -> Data Type Conversion19/1
  Data Type Conversion20/1 -> Shift Arithmetic22/1
  Shift Arithmetic22/1 -> Bitwise Operator/8
  Md27IsTargetPosAlready/1 -> Data Type Conversion20/1
  Data Type Conversion21/1 -> Shift Arithmetic23/1
  Md27IsTargetPosZone/1 -> Data Type Conversion21/1
  Shift Arithmetic23/1 -> Bitwise Operator1/8

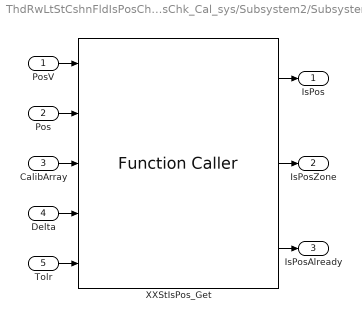
== system ThdRwLtStCshnFldIsPosChk1/ThdRwLtStCshnFldIsPosChk_Cal_sys/Subsystem2/Subsystem2 ==
  PosV : Inport
  Pos : Inport  Port=2
  CalibArray : Inport  Port=3
  Delta : Inport  Port=4
  Tolr : Inport  Port=5
  XXStIsPos_Get : FunctionCaller  FunctionPrototype=[IsPos,IsPosZone,IsPosAlready] = XXStIsPos_Get(PosV,Pos,CalibArray,Delta,Tolr)  InputArgumentSpecifications=boolean(true), uint16(1), uint16([1;1;1]), uint16(1), uint16(1)  OutputArgumentSpecifications=boolean(true), boolean(true), boolean(true)
  IsPos : Outport  VectorParamsAs1DForOutWhenUnconnected=off
  IsPosZone : Outport  Port=2  VectorParamsAs1DForOutWhenUnconnected=off
  IsPosAlready : Outport  Port=3  VectorParamsAs1DForOutWhenUnconnected=off
  wires:
  Pos/1 -> XXStIsPos_Get/2
  Delta/1 -> XXStIsPos_Get/4
  CalibArray/1 -> XXStIsPos_Get/3
  XXStIsPos_Get/2 -> IsPosZone/1
  XXStIsPos_Get/1 -> IsPos/1
  Tolr/1 -> XXStIsPos_Get/5
  XXStIsPos_Get/3 -> IsPosAlready/1
  PosV/1 -> XXStIsPos_Get/1

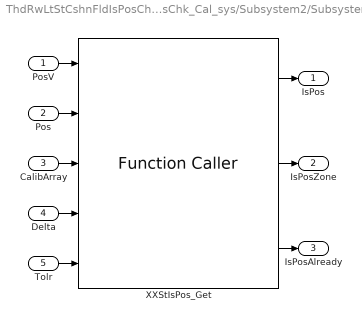
== system ThdRwLtStCshnFldIsPosChk1/ThdRwLtStCshnFldIsPosChk_Cal_sys/Subsystem2/Subsystem3 ==
  PosV : Inport
  Pos : Inport  Port=2
  CalibArray : Inport  Port=3
  Delta : Inport  Port=4
  Tolr : Inport  Port=5
  XXStIsPos_Get : FunctionCaller  FunctionPrototype=[IsPos,IsPosZone,IsPosAlready] = XXStIsPos_Get(PosV,Pos,CalibArray,Delta,Tolr)  InputArgumentSpecifications=boolean(true), uint16(1), uint16([1;1;1]), uint16(1), uint16(1)  OutputArgumentSpecifications=boolean(true), boolean(true), boolean(true)
  IsPos : Outport  VectorParamsAs1DForOutWhenUnconnected=off
  IsPosZone : Outport  Port=2  VectorParamsAs1DForOutWhenUnconnected=off
  IsPosAlready : Outport  Port=3  VectorParamsAs1DForOutWhenUnconnected=off
  wires:
  PosV/1 -> XXStIsPos_Get/1
  XXStIsPos_Get/3 -> IsPosAlready/1
  Tolr/1 -> XXStIsPos_Get/5
  XXStIsPos_Get/1 -> IsPos/1
  XXStIsPos_Get/2 -> IsPosZone/1
  CalibArray/1 -> XXStIsPos_Get/3
  Delta/1 -> XXStIsPos_Get/4
  Pos/1 -> XXStIsPos_Get/2

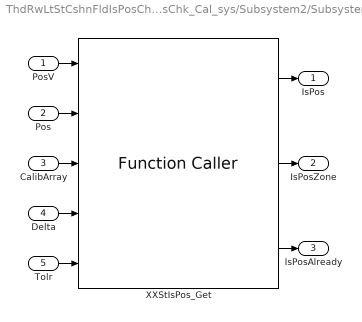
== system ThdRwLtStCshnFldIsPosChk1/ThdRwLtStCshnFldIsPosChk_Cal_sys/Subsystem2/Subsystem4 ==
  PosV : Inport
  Pos : Inport  Port=2
  CalibArray : Inport  Port=3
  Delta : Inport  Port=4
  Tolr : Inport  Port=5
  XXStIsPos_Get : FunctionCaller  FunctionPrototype=[IsPos,IsPosZone,IsPosAlready] = XXStIsPos_Get(PosV,Pos,CalibArray,Delta,Tolr)  InputArgumentSpecifications=boolean(true), uint16(1), uint16([1;1;1]), uint16(1), uint16(1)  OutputArgumentSpecifications=boolean(true), boolean(true), boolean(true)
  IsPos : Outport  VectorParamsAs1DForOutWhenUnconnected=off
  IsPosZone : Outport  Port=2  VectorParamsAs1DForOutWhenUnconnected=off
  IsPosAlready : Outport  Port=3  VectorParamsAs1DForOutWhenUnconnected=off
  wires:
  PosV/1 -> XXStIsPos_Get/1
  XXStIsPos_Get/3 -> IsPosAlready/1
  Tolr/1 -> XXStIsPos_Get/5
  XXStIsPos_Get/1 -> IsPos/1
  XXStIsPos_Get/2 -> IsPosZone/1
  CalibArray/1 -> XXStIsPos_Get/3
  Delta/1 -> XXStIsPos_Get/4
  Pos/1 -> XXStIsPos_Get/2

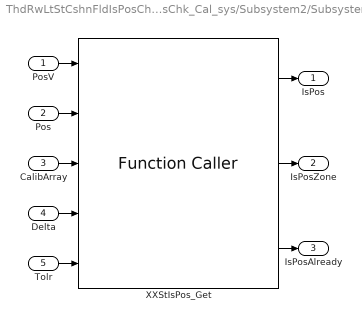
== system ThdRwLtStCshnFldIsPosChk1/ThdRwLtStCshnFldIsPosChk_Cal_sys/Subsystem2/Subsystem5 ==
  PosV : Inport
  Pos : Inport  Port=2
  CalibArray : Inport  Port=3
  Delta : Inport  Port=4
  Tolr : Inport  Port=5
  XXStIsPos_Get : FunctionCaller  FunctionPrototype=[IsPos,IsPosZone,IsPosAlready] = XXStIsPos_Get(PosV,Pos,CalibArray,Delta,Tolr)  InputArgumentSpecifications=boolean(true), uint16(1), uint16([1;1;1]), uint16(1), uint16(1)  OutputArgumentSpecifications=boolean(true), boolean(true), boolean(true)
  IsPos : Outport  VectorParamsAs1DForOutWhenUnconnected=off
  IsPosZone : Outport  Port=2  VectorParamsAs1DForOutWhenUnconnected=off
  IsPosAlready : Outport  Port=3  VectorParamsAs1DForOutWhenUnconnected=off
  wires:
  Pos/1 -> XXStIsPos_Get/2
  Delta/1 -> XXStIsPos_Get/4
  CalibArray/1 -> XXStIsPos_Get/3
  XXStIsPos_Get/2 -> IsPosZone/1
  XXStIsPos_Get/1 -> IsPos/1
  Tolr/1 -> XXStIsPos_Get/5
  XXStIsPos_Get/3 -> IsPosAlready/1
  PosV/1 -> XXStIsPos_Get/1

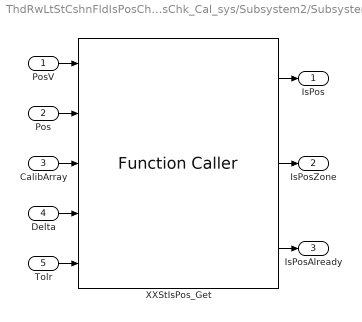
== system ThdRwLtStCshnFldIsPosChk1/ThdRwLtStCshnFldIsPosChk_Cal_sys/Subsystem2/Subsystem6 ==
  PosV : Inport
  Pos : Inport  Port=2
  CalibArray : Inport  Port=3
  Delta : Inport  Port=4
  Tolr : Inport  Port=5
  XXStIsPos_Get : FunctionCaller  FunctionPrototype=[IsPos,IsPosZone,IsPosAlready] = XXStIsPos_Get(PosV,Pos,CalibArray,Delta,Tolr)  InputArgumentSpecifications=boolean(true), uint16(1), uint16([1;1;1]), uint16(1), uint16(1)  OutputArgumentSpecifications=boolean(true), boolean(true), boolean(true)
  IsPos : Outport  VectorParamsAs1DForOutWhenUnconnected=off
  IsPosZone : Outport  Port=2  VectorParamsAs1DForOutWhenUnconnected=off
  IsPosAlready : Outport  Port=3  VectorParamsAs1DForOutWhenUnconnected=off
  wires:
  PosV/1 -> XXStIsPos_Get/1
  XXStIsPos_Get/3 -> IsPosAlready/1
  Tolr/1 -> XXStIsPos_Get/5
  XXStIsPos_Get/1 -> IsPos/1
  XXStIsPos_Get/2 -> IsPosZone/1
  CalibArray/1 -> XXStIsPos_Get/3
  Delta/1 -> XXStIsPos_Get/4
  Pos/1 -> XXStIsPos_Get/2

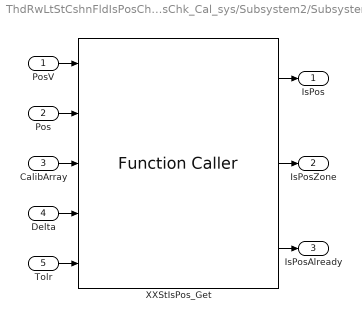
== system ThdRwLtStCshnFldIsPosChk1/ThdRwLtStCshnFldIsPosChk_Cal_sys/Subsystem2/Subsystem7 ==
  PosV : Inport
  Pos : Inport  Port=2
  CalibArray : Inport  Port=3
  Delta : Inport  Port=4
  Tolr : Inport  Port=5
  XXStIsPos_Get : FunctionCaller  FunctionPrototype=[IsPos,IsPosZone,IsPosAlready] = XXStIsPos_Get(PosV,Pos,CalibArray,Delta,Tolr)  InputArgumentSpecifications=boolean(true), uint16(1), uint16([1;1;1]), uint16(1), uint16(1)  OutputArgumentSpecifications=boolean(true), boolean(true), boolean(true)
  IsPos : Outport  VectorParamsAs1DForOutWhenUnconnected=off
  IsPosZone : Outport  Port=2  VectorParamsAs1DForOutWhenUnconnected=off
  IsPosAlready : Outport  Port=3  VectorParamsAs1DForOutWhenUnconnected=off
  wires:
  Pos/1 -> XXStIsPos_Get/2
  Delta/1 -> XXStIsPos_Get/4
  CalibArray/1 -> XXStIsPos_Get/3
  XXStIsPos_Get/2 -> IsPosZone/1
  XXStIsPos_Get/1 -> IsPos/1
  Tolr/1 -> XXStIsPos_Get/5
  XXStIsPos_Get/3 -> IsPosAlready/1
  PosV/1 -> XXStIsPos_Get/1

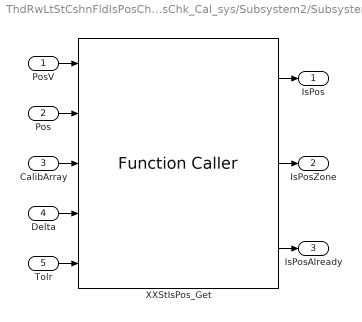
== system ThdRwLtStCshnFldIsPosChk1/ThdRwLtStCshnFldIsPosChk_Cal_sys/Subsystem2/Subsystem8 ==
  PosV : Inport
  Pos : Inport  Port=2
  CalibArray : Inport  Port=3
  Delta : Inport  Port=4
  Tolr : Inport  Port=5
  XXStIsPos_Get : FunctionCaller  FunctionPrototype=[IsPos,IsPosZone,IsPosAlready] = XXStIsPos_Get(PosV,Pos,CalibArray,Delta,Tolr)  InputArgumentSpecifications=boolean(true), uint16(1), uint16([1;1;1]), uint16(1), uint16(1)  OutputArgumentSpecifications=boolean(true), boolean(true), boolean(true)
  IsPos : Outport  VectorParamsAs1DForOutWhenUnconnected=off
  IsPosZone : Outport  Port=2  VectorParamsAs1DForOutWhenUnconnected=off
  IsPosAlready : Outport  Port=3  VectorParamsAs1DForOutWhenUnconnected=off
  wires:
  Pos/1 -> XXStIsPos_Get/2
  Delta/1 -> XXStIsPos_Get/4
  CalibArray/1 -> XXStIsPos_Get/3
  XXStIsPos_Get/2 -> IsPosZone/1
  XXStIsPos_Get/1 -> IsPos/1
  Tolr/1 -> XXStIsPos_Get/5
  XXStIsPos_Get/3 -> IsPosAlready/1
  PosV/1 -> XXStIsPos_Get/1
